simulink library "lib_HVESS"  (R2017a)
settings: Solver=VariableStepAuto  StartTime=0.0  StopTime=10.0  RelTol=1e-3
undefined symbols (not defined in the file): Atm_temp, bms_inletair_temp, bms_maxchargecurrent, bms_maxdischargecurrent, BMS_Notfallkuehlung, Cells, Chg, Em, ess, I_loss, mph2kph, R_0, R_1, SOC_bp, T_bp, tloop
libraries: fl_lib x13, simulink x9, nesl_utility x8, RollingAliveCounter x1
(part 1 of 2)
settings Model: Creator=Di Russo  LastModifiedBy=Vraj M

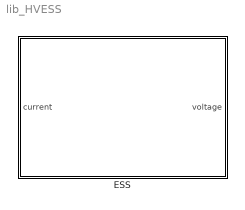
== system lib_HVESS ==
  ESS : Subsystem
      mask Display:
      | image('Images/ESS.jpg')
      | color('red');
      | port_label('Input',1,'Crr');
      | port_label('Output',1,'Volt');

== system lib_HVESS/ESS ==
  note: BMS_to_Actuators
  current : Inport
  ESS : Subsystem
      mask Display:
      | image('Images/ESS.jpg')
      | color('red');
      | port_label('Input',2,'Crr');
      | port_label('Output',2,'Volt');
  Inputs : Subsystem
  Outputs : Subsystem
  Soft BMS : Subsystem  RequirementInfo={} %GIDa_db9a4bec_736d_475e_b698_7a828f195e96
      mask Display: image('SoftECU.jpg')
  voltage : Outport
  wires:
  Inputs/1(Inputs) -> Soft BMS/1(Input1)
  Soft BMS/1(CAN) -> Outputs/1(Outputs)
  ESS/2(Voltage) -> voltage/1
  ESS/1(out) -> Soft BMS/2(Input2)  "Sensors_to_BMS"
  Soft BMS/2(Output2) -> ESS/1("In ")
  current/1 -> ESS/2("Crr ")

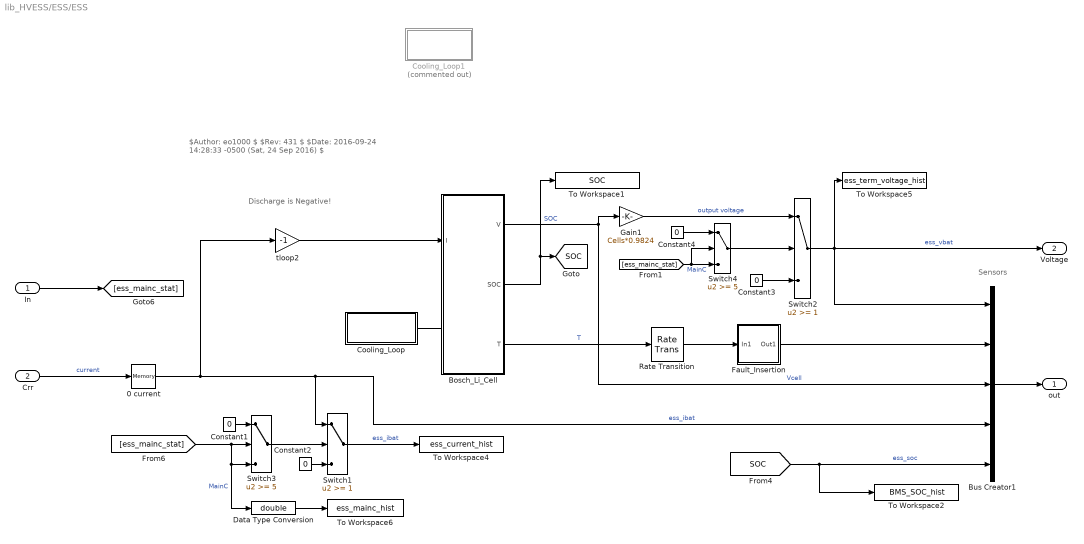
== system lib_HVESS/ESS/ESS ==
  note: $Author: eo1000 $
      | $Rev: 431 $
      | $Date: 2016-09-24 14:28:33 -0500 (Sat, 24 Sep 2016) $
  note: Discharge is Negative!
  note: Sensors
  "In " : Inport
  "Crr " : Inport  Port=2
  0 current : Memory  InheritSampleTime=on
  Bosch_Li_Cell : Subsystem
  Bus Creator1 : BusCreator  Inputs=5
  Constant{1..4} (4 alike) : Constant  Value=0
  Cooling_Loop : Subsystem
  Cooling_Loop1 : Subsystem  Commented=on
  Data Type Conversion : DataTypeConversion  OutDataTypeStr=double
  Fault_Insertion : Subsystem
  Gain1 : Gain  Gain=Cells*0.9824
  Rate Transition : RateTransition  X0=273.15+25
  Switch1 : Switch  Threshold=1
  Switch2 : Switch  Threshold=1
  Switch3 : Switch  Threshold=5
  Switch4 : Switch  Threshold=5
  To Workspace1 : ToWorkspace  VariableName=SOC  SampleTime=-1
      settings: Decimation=WORKSPACE_DECIMATION
  To Workspace2 : ToWorkspace  VariableName=BMS_SOC_hist  SampleTime=-1
      settings: Decimation=WORKSPACE_DECIMATION
  To Workspace4 : ToWorkspace  VariableName=ess_current_hist  SampleTime=-1
      settings: Decimation=WORKSPACE_DECIMATION
  To Workspace5 : ToWorkspace  VariableName=ess_term_voltage_hist  SampleTime=-1
      settings: Decimation=WORKSPACE_DECIMATION
  To Workspace6 : ToWorkspace  VariableName=ess_mainc_hist  SampleTime=-1
      settings: Decimation=WORKSPACE_DECIMATION
  tloop2 : Gain  Gain=-1
  out : Outport
  Voltage : Outport  Port=2
  tag scope: SOC=global
  wires:
  Rate Transition/1 -> Fault_Insertion/1(In1)
  Fault_Insertion/1(Out1) -> Bus Creator1/2
  tloop2/1 -> Bosch_Li_Cell/1(I)
  Bosch_Li_Cell/2(SOC) -> [SOC], To Workspace1/1  "SOC"
  Bosch_Li_Cell/3(T) -> Rate Transition/1  "T"
  "Crr "/1 -> 0 current/1  "current"
  0 current/1 -> Switch1/1, Bus Creator1/4, tloop2/1  "ess_ibat"
  Switch4/1 -> Switch2/2
  Constant4/1 -> Switch4/1
  [ess_mainc_stat] -> Switch4/2, Switch4/3  "MainC"
  Switch3/1 -> Switch1/2
  Constant1/1 -> Switch3/1
  Bosch_Li_Cell/1(V) -> Bus Creator1/3, Gain1/1  "Vcell"
  [SOC] -> Bus Creator1/5, To Workspace2/1  "ess_soc"
  Switch2/1 -> To Workspace5/1, Voltage/1, Bus Creator1/1  "ess_vbat"
  Constant3/1 -> Switch2/3
  [ess_mainc_stat] -> Switch3/2, Switch3/3, Data Type Conversion/1  "MainC"
  Gain1/1 -> Switch2/1  "output voltage"
  Switch1/1 -> To Workspace4/1  "ess_ibat"
  Constant2/1 -> Switch1/3
  Data Type Conversion/1 -> To Workspace6/1
  Bus Creator1/1 -> out/1
  "In "/1 -> [ess_mainc_stat]
  connections:
  Cooling_Loop/RConn1 -- Bosch_Li_Cell/LConn1

== system lib_HVESS/ESS/Inputs ==
  Bus Creator1 : BusCreator  Inputs=2
  CAN_fromHCU : Subsystem
  Digital_fromHCU : Subsystem
  Inputs : Outport
  wires:
  Bus Creator1/1 -> Inputs/1
  CAN_fromHCU/1(Outputs) -> Bus Creator1/1  "CAN"
  Digital_fromHCU/1(Outputs) -> Bus Creator1/2  "Digital"

== system lib_HVESS/ESS/Outputs ==
  Outputs : Inport
  tag scope: BMS_to_HCU=global
  wires:
  Outputs/1 -> [BMS_to_HCU]  "BMS_CAN"

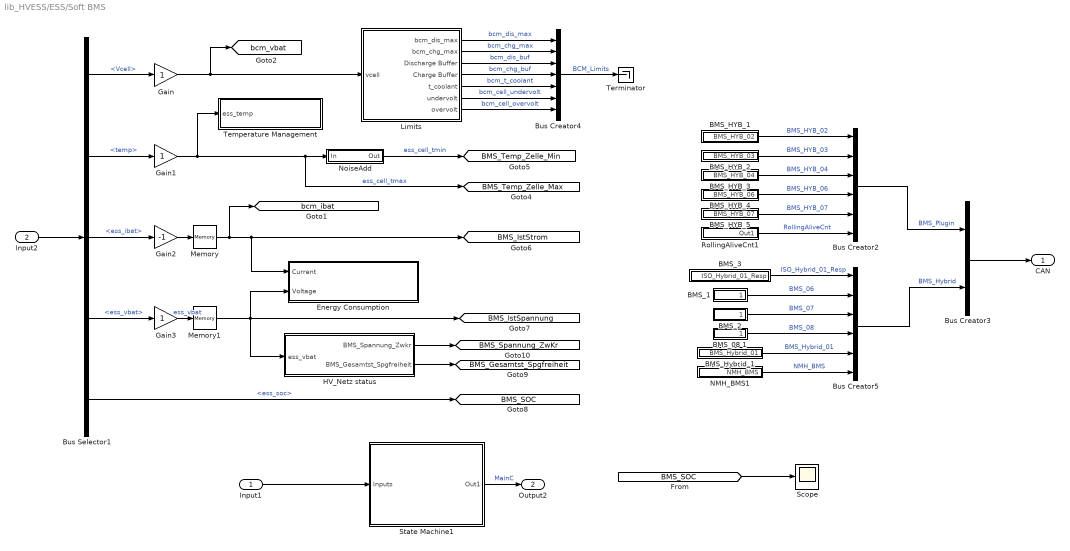
== system lib_HVESS/ESS/Soft BMS ==
  Input1 : Inport
  Input2 : Inport  Port=2
  BMS_08 1 : Subsystem
  BMS_1 : Subsystem
  BMS_2 : Subsystem
  BMS_3 : Subsystem
  BMS_HYB_1 : Subsystem
  BMS_HYB_2 : Subsystem
  BMS_HYB_3 : Subsystem
  BMS_HYB_4 : Subsystem
  BMS_HYB_5 : Subsystem
  BMS_Hybrid_1 : Subsystem
  Bus Creator2 : BusCreator  Inputs=6
  Bus Creator3 : BusCreator  Inputs=2
  Bus Creator4 : BusCreator  Inputs=7
  Bus Creator5 : BusCreator  Inputs=6
  Bus Selector1 : BusSelector  OutputSignals=Vcell,temp,ess_ibat,ess_vbat,ess_soc
  Energy Consumption : Subsystem
  Gain : Gain
  Gain1 : Gain
  Gain2 : Gain  Gain=-1
  Gain3 : Gain
  HV_Netz status : Subsystem
  Limits : Subsystem
  Memory : Memory
  Memory1 : Memory
  NMH_BMS1 : Subsystem
  NoiseAdd : Subsystem
  RollingAliveCnt1 : Subsystem
  Scope : Scope
  State Machine1 : Subsystem
  Temperature Management : Subsystem
  Terminator : Terminator
  CAN : Outport
  Output2 : Outport  Port=2
  tag scope: BMS_Gesamtst_Spgfreiheit=global, BMS_IstSpannung=global, BMS_IstStrom=global, BMS_SOC=global, BMS_Spannung_ZwKr=global, BMS_Temp_Zelle_Max=global, BMS_Temp_Zelle_Min=global, bcm_ibat=global, bcm_vbat=global
  wires:
  [BMS_SOC] -> Scope/1
  RollingAliveCnt1/1(Out1) -> Bus Creator2/6  "RollingAliveCnt"
  BMS_3/1(ISO_Hybrid_01_Resp) -> Bus Creator5/1  "ISO_Hybrid_01_Resp"
  Bus Creator2/1 -> Bus Creator3/1  "BMS_Plugin"
  Bus Creator5/1 -> Bus Creator3/2  "BMS_Hybrid"
  BMS_08 1/1(BMS_08) -> Bus Creator5/4  "BMS_08"
  BMS_1/1(BMS_06) -> Bus Creator5/2  "BMS_06"
  BMS_HYB_4/1(BMS_HYB_06) -> Bus Creator2/4  "BMS_HYB_06"
  BMS_HYB_1/1(BMS_HYB_02) -> Bus Creator2/1  "BMS_HYB_02"
  BMS_HYB_3/1(BMS_HYB_04) -> Bus Creator2/3  "BMS_HYB_04"
  BMS_2/1(BMS_07) -> Bus Creator5/3  "BMS_07"
  BMS_Hybrid_1/1(BMS_Hybrid_01) -> Bus Creator5/5  "BMS_Hybrid_01"
  BMS_HYB_5/1(BMS_HYB_07) -> Bus Creator2/5  "BMS_HYB_07"
  BMS_HYB_2/1(BMS_HYB_03) -> Bus Creator2/2  "BMS_HYB_03"
  NMH_BMS1/1(NMH_BMS) -> Bus Creator5/6  "NMH_BMS"
  Memory1/1 -> Energy Consumption/2(Voltage), HV_Netz status/1(ess_vbat), [BMS_IstSpannung]
  Memory/1 -> [BMS_IstStrom], Energy Consumption/1(Current), [bcm_ibat]
  HV_Netz status/2(BMS_Gesamtst_Spgfreiheit) -> [BMS_Gesamtst_Spgfreiheit]
  HV_Netz status/1(BMS_Spannung_Zwkr) -> [BMS_Spannung_ZwKr]
  Bus Creator3/1 -> CAN/1
  Limits/7(overvolt) -> Bus Creator4/7  "bcm_cell_overvolt"
  Limits/6(undervolt) -> Bus Creator4/6  "bcm_cell_undervolt"
  Bus Selector1/4 -> Gain3/1  "<ess_vbat>"
  Bus Selector1/5 -> [BMS_SOC]  "<ess_soc>"
  Bus Creator4/1 -> Terminator/1  "BCM_Limits"
  Limits/2(bcm_chg_max) -> Bus Creator4/2  "bcm_chg_max"
  Limits/5(t_coolant) -> Bus Creator4/5  "bcm_t_coolant"
  Limits/4(Charge Buffer) -> Bus Creator4/4  "bcm_chg_buf"
  Limits/3(Discharge Buffer) -> Bus Creator4/3  "bcm_dis_buf"
  Limits/1(bcm_dis_max) -> Bus Creator4/1  "bcm_dis_max"
  Gain1/1 -> [BMS_Temp_Zelle_Max], NoiseAdd/1(In), Temperature Management/1(ess_temp)  "ess_cell_tmax"
  Bus Selector1/2 -> Gain1/1  "<temp>"
  Bus Selector1/1 -> Gain/1  "<Vcell>"
  NoiseAdd/1(Out) -> [BMS_Temp_Zelle_Min]  "ess_cell_tmin"
  Bus Selector1/3 -> Gain2/1  "<ess_ibat>"
  Input2/1 -> Bus Selector1/1
  Input1/1 -> State Machine1/1(Inputs)
  Gain/1 -> Limits/1(vcell), [bcm_vbat]
  Gain2/1 -> Memory/1
  Gain3/1 -> Memory1/1  "ess_vbat"
  State Machine1/1(Out1) -> Output2/1  "MainC"

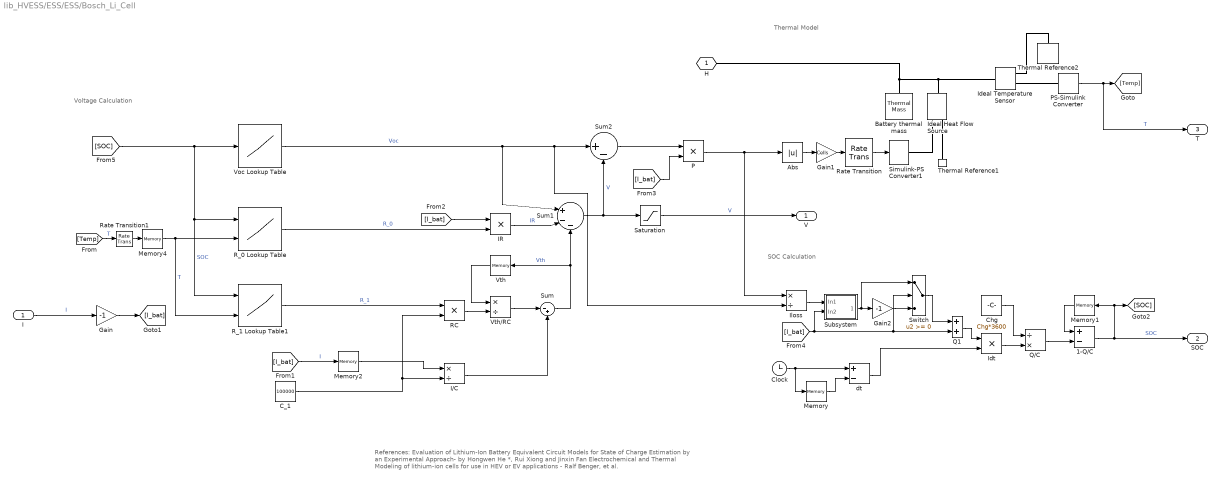
== system lib_HVESS/ESS/ESS/Bosch_Li_Cell ==
  note: SOC Calculation
  note: Thermal Model
  note: Voltage Calculation
  note: References:
      | Evaluation of Lithium-Ion Battery Equivalent Circuit Models for State of Charge Estimation by an Experimental Approach- by Hongwen He *, Rui Xiong and Jinxin Fan
      | Electrochemical and Thermal Modeling of lithium-ion cells for use in HEV or EV applications - Ralf Benger, et al.
  I : Inport
  1-Q/C : Sum  Inputs=+-
  Abs : Abs
  Battery thermal mass : fl_lib/Thermal/Thermal Elements/Thermal Mass  mass=155 kg  sp_heat=800 J/kg/K  T_specify=off  T_priority=High  T=Atm_temp degC  T_nominal_specify=off  T_nominal_unit=K  T_nominal_value=1  Q_specify=off  Q_priority=High  Q=0 J/s  Q_nominal_specify=off  Q_nominal_unit=J/s  Q_nominal_value=1
  C_1 : Constant  Value=100000
  Chg : Constant  Value=Chg*3600
  Clock : Clock
  Gain : Gain  Gain=-1
  Gain1 : Gain  Gain=Cells
  Gain2 : Gain  Gain=-1
  I/C : Product  Inputs=*/
  IR : Product  Inputs=**
  Ideal Heat Flow Source : fl_lib/Thermal/Thermal Sources/Ideal Heat Flow Source
      settings: SourceProductName=Simscape  SourceProductBaseCode=SS
  Ideal Temperature Sensor : fl_lib/Thermal/Thermal Sensors/Ideal Temperature Sensor
      settings: SourceProductName=Simscape  SourceProductBaseCode=SS
  Idt : Product  Inputs=**
  Iloss : Product  Inputs=*/
  Memory : Memory  InheritSampleTime=on
  Memory1 : Memory  X0=ess.plant.initial_soc/100  InheritSampleTime=on
  Memory2 : Memory  InheritSampleTime=on
  Memory4 : Memory  X0=298
  P : Product  Inputs=**
  PS-Simulink Converter : nesl_utility/PS-Simulink Converter  PhysicalDomain=network_engine_domain  SubClassName=ps_output  LeftPortType=input  RightPortType=output  PseudoPeriodic=off  Frequencies=[]  Unit=1  AffineConversion=off
  Q/C : Product  Inputs=/*
  Q1 : Sum
  RC : Product  Inputs=**
  R_0 Lookup Table : Lookup_n-D  BreakpointsForDimension1=SOC_bp  BreakpointsForDimension2=T_bp  Table=R_0  UseLastTableValue=on  InternalRulePriority=Speed  RndMeth=Simplest  InputSameDT=on
  R_1 Lookup Table1 : Lookup_n-D  BreakpointsForDimension1=SOC_bp  BreakpointsForDimension2=T_bp  Table=R_1  UseLastTableValue=on  InternalRulePriority=Speed  RndMeth=Simplest  InputSameDT=on
  Rate Transition : RateTransition
  Rate Transition1 : RateTransition
  Saturation : Saturate  UpperLimit=4.2  LowerLimit=2.8
  Simulink-PS Converter1 : nesl_utility/Simulink-PS Converter  PhysicalDomain=network_engine_domain  SubClassName=ps_input  LeftPortType=input  RightPortType=output  PseudoPeriodic=off  Frequencies=[]  NoiseDistribution=none  NoiseParameters=[]  Unit=1  AffineConversion=off  FilteringAndDerivatives=zero  SimscapeFilterOrder=1  InputFilterTimeConstant=0.001  UdotUserProvided=1
  Subsystem : Subsystem
  Sum : Sum  Inputs=|-+
  Sum1 : Sum  Inputs=|+--
  Sum2 : Sum  Inputs=|+-
  Switch : Switch
  Thermal Reference1 : fl_lib/Thermal/Thermal Elements/Thermal Reference
  Thermal Reference2 : fl_lib/Thermal/Thermal Elements/Thermal Reference
  Voc Lookup Table : Lookup_n-D  NumberOfTableDimensions=1  BreakpointsForDimension1=SOC_bp  Table=Em  InternalRulePriority=Speed  RndMeth=Simplest  InputSameDT=on
  Vth : Memory  InheritSampleTime=on  LinearizeAsDelay=on
  Vth/RC : Product  Inputs=*/
  dt : Sum  Inputs=+-
  H : PMIOPort  Tag=PMCPort  Port=1  Side=Left
  V : Outport
  SOC : Outport  Port=2
  T : Outport  Port=3
  wires:
  Rate Transition1/1 -> Memory4/1
  Subsystem/1(Out1) -> Gain2/1, Switch/1
  Iloss/1 -> Subsystem/1(In1)
  Switch/1 -> Q1/1
  Q1/1 -> Idt/1
  Gain2/1 -> Switch/3
  Gain1/1 -> Rate Transition/1
  P/1 -> Abs/1, Iloss/1
  Memory2/1 -> I/C/1
  Idt/1 -> Q/C/2
  dt/1 -> Idt/2
  Memory/1 -> dt/2
  Clock/1 -> dt/1, Memory/1
  Gain/1 -> [I_bat]
  Memory1/1 -> 1-Q/C/1
  Q/C/1 -> 1-Q/C/2
  Chg/1 -> Q/C/1
  1-Q/C/1 -> [SOC], Memory1/1, SOC/1  "SOC"
  Memory4/1 -> R_0 Lookup Table/2, R_1 Lookup Table1/2  "T"
  Saturation/1 -> V/1  "V"
  I/1 -> Gain/1  "I"
  Voc Lookup Table/1 -> Sum1/1, Sum2/1, Iloss/2  "Voc"
  R_1 Lookup Table1/1 -> RC/1  "R_1"
  PS-Simulink Converter/1 -> [Temp], T/1  "T"
  [I_bat] -> P/2
  [I_bat] -> IR/1
  Sum1/1 -> Sum2/2, Saturation/1  "V"
  Vth/1 -> Vth/RC/1
  I/C/1 -> Sum/2
  [I_bat] -> Memory2/1  "I"
  RC/1 -> Vth/RC/2
  C_1/1 -> I/C/2, RC/2
  Sum2/1 -> P/1
  Sum/1 -> Vth/1, Sum1/3  "Vth"
  IR/1 -> Sum1/2  "IR"
  [SOC] -> Voc Lookup Table/1, R_1 Lookup Table1/1, R_0 Lookup Table/1  "SOC"
  [Temp] -> Rate Transition1/1  "T"
  Rate Transition/1 -> Simulink-PS Converter1/1
  Abs/1 -> Gain1/1
  [I_bat] -> Switch/2, Q1/2, Subsystem/2(In2)
  R_0 Lookup Table/1 -> IR/2  "R_0"
  Vth/RC/1 -> Sum/1
  connections:
  Ideal Heat Flow Source/RConn1 -- Simulink-PS Converter1/RConn1
  Ideal Temperature Sensor/RConn2 -- PS-Simulink Converter/LConn1
  Ideal Temperature Sensor/RConn1 -- Thermal Reference2/LConn1
  Ideal Heat Flow Source/RConn2 -- Thermal Reference1/LConn1
  Ideal Heat Flow Source/LConn1 -- Battery thermal mass/LConn1 -- H/RConn1 -- Ideal Temperature Sensor/LConn1

== system lib_HVESS/ESS/ESS/Cooling_Loop ==
  Constant : Constant  Value=Atm_temp+273+0.5
  Convective Heat Transfer : fl_lib/Thermal/Thermal Elements/Convective Heat Transfer  area=1e-4*Cells*0.25 m^2  heat_tr_coeff=H_coef W/(m^2 * K)  Q_specify=off  Q_priority=High  Q=0 J/s  Q_nominal_specify=off  Q_nominal_unit=J/s  Q_nominal_value=1  T_specify=off  T_priority=High  T=0 K  T_nominal_specify=off  T_nominal_unit=K  T_nominal_value=1
  Ideal Temperature Source : fl_lib/Thermal/Thermal Sources/Ideal Temperature Source
      settings: SourceProductName=Simscape  SourceProductBaseCode=SS
  Simulink-PS Converter : nesl_utility/Simulink-PS Converter  PhysicalDomain=network_engine_domain  SubClassName=ps_input  LeftPortType=input  RightPortType=output  PseudoPeriodic=off  Frequencies=[]  NoiseDistribution=none  NoiseParameters=[]  Unit=1  AffineConversion=off  FilteringAndDerivatives=zero  SimscapeFilterOrder=1  InputFilterTimeConstant=0.001  UdotUserProvided=1
  Solver Configuration : nesl_utility/Solver Configuration  PhysicalDomain=network_engine_domain  SubClassName=solver  LeftPortType=input  RightPortType=generic  Accelerate=off  Tones=[]  Harmonics=[]  SimulateNoise=off  Profile=off  UseLocalSampling=off  EnableSwitchedLinearOptims=on  FrequencyDomain=off  UseCCode=off  RelTol=0.001  AbsTol=1e-06  MinStep=1e-09  ToWorkspace=off  RevertToSquareIcSolve=off  NumHomotopyIterations=100  PhasorMode=off  PhasorModeNumHarmonics=1  OverrideAbsTol=off  DoDC=off  ResidualTolerance=1e-09  UseLocalSolver=on  LocalSolverChoice=NE_TRAPEZOIDAL_ADVANCER  LocalSolverSampleTime=1  DoFixedCost=on  MaxNonlinIter=3  MaxModeIter=2  LinearAlgebra=Sparse  DelaysMemoryBudget=1024  AutomaticFiltering=on  FilteringTimeConstant=0.001
  Thermal Reference : fl_lib/Thermal/Thermal Elements/Thermal Reference
  Conn1 : PMIOPort  Port=1  Side=Right
  wires:
  Constant/1 -> Simulink-PS Converter/1
  connections:
  Conn1/RConn1 -- Solver Configuration/RConn1 -- Convective Heat Transfer/LConn1
  Ideal Temperature Source/RConn1 -- Simulink-PS Converter/RConn1
  Ideal Temperature Source/LConn1 -- Convective Heat Transfer/RConn1
  Ideal Temperature Source/RConn2 -- Thermal Reference/LConn1

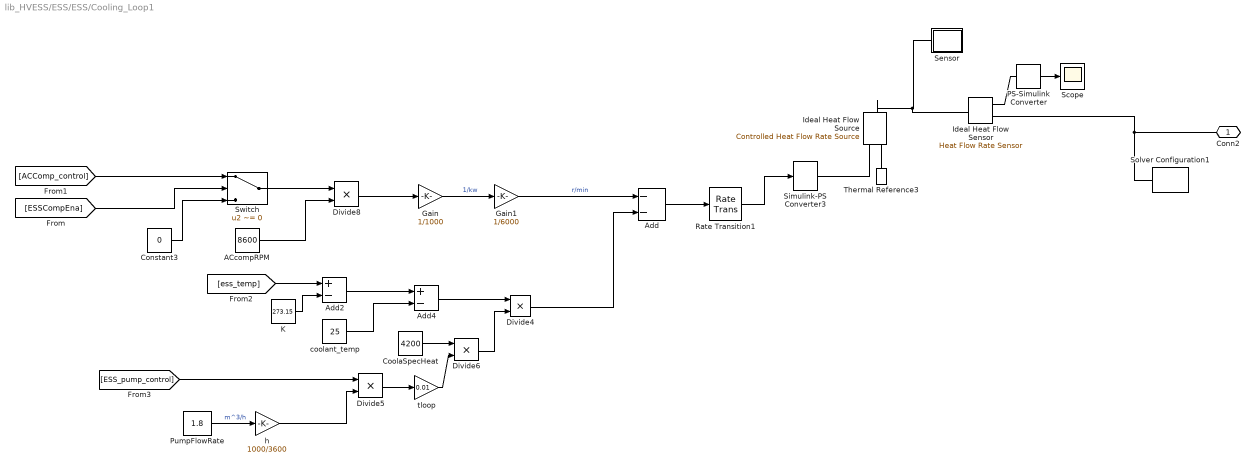
== system lib_HVESS/ESS/ESS/Cooling_Loop1 ==
  ACcompRPM : Constant  Value=8600
  Add : Sum  Inputs=--
  Add2 : Sum  Inputs=+-
  Add4 : Sum  Inputs=+-
  Constant3 : Constant  Value=0
  CoolaSpecHeat : Constant  Value=4200
  Divide{4..6,8} (4 alike) : Product  Inputs=**
  Gain : Gain  Gain=1/1000
  Gain1 : Gain  Gain=1/6000
  Ideal Heat Flow Sensor : fl_lib/Thermal/Thermal Sensors/Heat Flow Rate Sensor
      settings: SourceProductName=Simscape  SourceProductBaseCode=SS
  Ideal Heat Flow Source : fl_lib/Thermal/Thermal Sources/Controlled Heat Flow Rate Source
      settings: SourceProductName=Simscape
  K : Constant  Value=273.15
  PS-Simulink Converter : nesl_utility/PS-Simulink Converter  PhysicalDomain=network_engine_domain  SubClassName=ps_output  LeftPortType=input  RightPortType=output  PseudoPeriodic=off  Frequencies=[]  Unit=1  AffineConversion=off
  PumpFlowRate : Constant  Value=1.8
  Rate Transition1 : RateTransition
  Scope : Scope
  Sensor : Subsystem
  Simulink-PS Converter3 : nesl_utility/Simulink-PS Converter  PhysicalDomain=network_engine_domain  SubClassName=ps_input  LeftPortType=input  RightPortType=output  PseudoPeriodic=off  Frequencies=[]  NoiseDistribution=none  NoiseParameters=[]  Unit=J/s  AffineConversion=off  FilteringAndDerivatives=zero  SimscapeFilterOrder=1  InputFilterTimeConstant=0.001  UdotUserProvided=1
  Solver Configuration1 : nesl_utility/Solver Configuration  PhysicalDomain=network_engine_domain  SubClassName=solver  LeftPortType=input  RightPortType=generic  Accelerate=off  Tones=[]  Harmonics=[]  SimulateNoise=off  Profile=off  UseLocalSampling=off  EnableSwitchedLinearOptims=on  FrequencyDomain=off  UseCCode=off  RelTol=0.001  AbsTol=1e-06  MinStep=1e-09  ToWorkspace=off  RevertToSquareIcSolve=off  NumHomotopyIterations=100  PhasorMode=off  PhasorModeNumHarmonics=1  OverrideAbsTol=off  DoDC=off  ResidualTolerance=1e-09  UseLocalSolver=on  LocalSolverChoice=NE_BACKWARD_EULER_ADVANCER  LocalSolverSampleTime=1  DoFixedCost=on  MaxNonlinIter=3  MaxModeIter=2  LinearAlgebra=Sparse  DelaysMemoryBudget=1024  AutomaticFiltering=on  FilteringTimeConstant=0.001
  Switch : Switch  Criteria=u2 ~= 0
  Thermal Reference3 : fl_lib/Thermal/Thermal Elements/Thermal Reference
  coolant_temp : Constant  Value=25
  h : Gain  Gain=1000/3600
  tloop : Gain  Gain=0.01
  Conn2 : PMIOPort  Port=1  Side=Left
  wires:
  PS-Simulink Converter/1 -> Scope/1
  [ESS_pump_control] -> Divide5/1
  Switch/1 -> Divide8/1
  Add/1 -> Rate Transition1/1
  Rate Transition1/1 -> Simulink-PS Converter3/1
  K/1 -> Add2/2
  [ess_temp] -> Add2/1
  Add2/1 -> Add4/1
  Constant3/1 -> Switch/3
  Divide4/1 -> Add/2
  PumpFlowRate/1 -> h/1  "m^3/h"
  Divide5/1 -> tloop/1
  ACcompRPM/1 -> Divide8/2
  Gain1/1 -> Add/1  "r/min"
  [ACComp_control] -> Switch/1
  Gain/1 -> Gain1/1  "1/kw"
  h/1 -> Divide5/2
  coolant_temp/1 -> Add4/2
  CoolaSpecHeat/1 -> Divide6/1
  Add4/1 -> Divide4/1
  Divide8/1 -> Gain/1
  tloop/1 -> Divide6/2
  Divide6/1 -> Divide4/2
  [ESSCompEna] -> Switch/2
  connections:
  Ideal Heat Flow Sensor/RConn1 -- PS-Simulink Converter/LConn1
  Conn2/RConn1 -- Ideal Heat Flow Sensor/RConn2 -- Solver Configuration1/RConn1
  Thermal Reference3/LConn1 -- Ideal Heat Flow Source/RConn2
  Simulink-PS Converter3/RConn1 -- Ideal Heat Flow Source/RConn1
  Sensor/LConn1 -- Ideal Heat Flow Sensor/LConn1 -- Ideal Heat Flow Source/LConn1

== system lib_HVESS/ESS/ESS/Fault_Insertion ==
  In1 : Inport
  Gain : Gain  Gain=3
  Switch : Switch  Threshold=1
  Out1 : Outport
  wires:
  Gain/1 -> Switch/1
  Switch/1 -> Out1/1  "temp"
  In1/1 -> Switch/3, Gain/1
  [ESSOverTemp] -> Switch/2

== system lib_HVESS/ESS/Inputs/CAN_fromHCU ==
  Bus Creator : BusCreator  Inputs=2
  Outputs : Outport
  wires:
  Bus Creator/1 -> Outputs/1
  [HCU_to_EBCAN] -> Bus Creator/2
  [HCU_to_HV_CAN] -> Bus Creator/1

== system lib_HVESS/ESS/Inputs/Digital_fromHCU ==
  Outputs : Outport
  wires:
  [Digital] -> Outputs/1

== system lib_HVESS/ESS/Soft BMS/BMS_08 1 ==
  Bus Creator8 : BusCreator  Inputs=2
  BMS_08 : Outport
  wires:
  [BMS_Temp_Zelle_Max] -> Bus Creator8/1  "BMS_Temp_Zelle_Max"
  Bus Creator8/1 -> BMS_08/1  "BMS_08"
  [BMS_Temp_Zelle_Min] -> Bus Creator8/2  "BMS_Temp_Zelle_Min"

== system lib_HVESS/ESS/Soft BMS/BMS_1 ==
  Bus Creator8 : BusCreator  Inputs=1
  Constant2 : Constant  Value=0
  BMS_06 : Outport
  wires:
  Constant2/1 -> Bus Creator8/1  "BMS_SollVolumenStrom"
  Bus Creator8/1 -> BMS_06/1  "BMS_06"

== system lib_HVESS/ESS/Soft BMS/BMS_2 ==
  Bus Creator8 : BusCreator  Inputs=1
  BMS_07 : Outport
  wires:
  [BMS_Gesamtst_Spgfreiheit] -> Bus Creator8/1  "BMS_Gesamtst_Spgfreiheit"
  Bus Creator8/1 -> BMS_07/1  "BMS_07"

== system lib_HVESS/ESS/Soft BMS/BMS_3 ==
  Bus Creator8 : BusCreator  Inputs=3
  Constant : Constant  Value=255
  Constant1 : Constant  Value=254
  Data Type Conversion : DataTypeConversion
  ISO_Hybrid_01_Resp : Outport
  wires:
  [ISO_Hybrid_01_Req_Data_4] -> Data Type Conversion/1  "ISO_Hybrid_01_Resp_Data_4"
  Constant1/1 -> Bus Creator8/3  "ISO_Hybrid_01_Resp_Data_6"
  Constant/1 -> Bus Creator8/2  "ISO_Hybrid_01_Resp_Data_5"
  Data Type Conversion/1 -> Bus Creator8/1  "ISO_Hybrid_01_Resp_Data_4"
  Bus Creator8/1 -> ISO_Hybrid_01_Resp/1  "ISO_Hybrid_01_Resp"

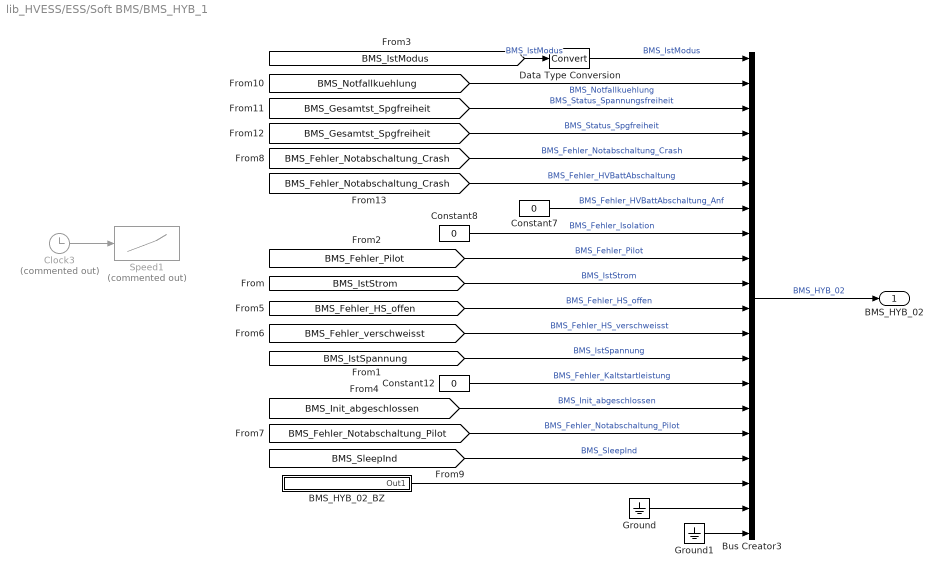
== system lib_HVESS/ESS/Soft BMS/BMS_HYB_1 ==
  BMS_HYB_02_BZ : Subsystem
  Bus Creator3 : BusCreator  Inputs=20
  Clock3 : Clock  Commented=on
  Constant12 : Constant  Value=0
  Constant7 : Constant  Value=0
  Constant8 : Constant  Value=0
  Data Type Conversion : DataTypeConversion
  Ground : Ground
  Ground1 : Ground
  Speed1 : Lookup  Commented=on  InputValues=[0 75 75 100 100 120]  Table=[0 0 1 1 0 0]
  BMS_HYB_02 : Outport
  wires:
  Ground1/1 -> Bus Creator3/20
  Ground/1 -> Bus Creator3/19
  BMS_HYB_02_BZ/1(Out1) -> Bus Creator3/18
  [BMS_IstModus] -> Data Type Conversion/1  "BMS_IstModus"
  Clock3/1 -> Speed1/1
  Bus Creator3/1 -> BMS_HYB_02/1  "BMS_HYB_02"
  Data Type Conversion/1 -> Bus Creator3/1  "BMS_IstModus"
  [BMS_Gesamtst_Spgfreiheit] -> Bus Creator3/3  "BMS_Status_Spannungsfreiheit"
  [BMS_Fehler_Notabschaltung_Crash] -> Bus Creator3/6  "BMS_Fehler_HVBattAbschaltung"
  Constant7/1 -> Bus Creator3/7  "BMS_Fehler_HVBattAbschaltung_Anf"
  [BMS_Notfallkuehlung] -> Bus Creator3/2  "BMS_Notfallkuehlung"
  Constant8/1 -> Bus Creator3/8  "BMS_Fehler_Isolation"
  [BMS_Fehler_Notabschaltung_Crash] -> Bus Creator3/5  "BMS_Fehler_Notabschaltung_Crash"
  [BMS_Gesamtst_Spgfreiheit] -> Bus Creator3/4  "BMS_Status_Spgfreiheit"
  [BMS_Fehler_Pilot] -> Bus Creator3/9  "BMS_Fehler_Pilot"
  [BMS_IstStrom] -> Bus Creator3/10  "BMS_IstStrom"
  [BMS_Fehler_HS_offen] -> Bus Creator3/11  "BMS_Fehler_HS_offen"
  [BMS_Fehler_verschweisst] -> Bus Creator3/12  "BMS_Fehler_HS_verschweisst"
  [BMS_IstSpannung] -> Bus Creator3/13  "BMS_IstSpannung"
  Constant12/1 -> Bus Creator3/14  "BMS_Fehler_Kaltstartleistung"
  [BMS_Init_abgeschlossen] -> Bus Creator3/15  "BMS_Init_abgeschlossen"
  [BMS_Fehler_Notabschaltung_Pilot] -> Bus Creator3/16  "BMS_Fehler_Notabschaltung_Pilot"
  [BMS_SleepInd] -> Bus Creator3/17  "BMS_SleepInd"

== system lib_HVESS/ESS/Soft BMS/BMS_HYB_2 ==
  Bus Creator3 : BusCreator  Inputs=1
  Data Type Conversion : DataTypeConversion
  Gain : Gain  Gain=100
  BMS_HYB_03 : Outport
  wires:
  Gain/1 -> Data Type Conversion/1
  [BMS_SOC] -> Gain/1  "BMS_SOC"
  Data Type Conversion/1 -> Bus Creator3/1  "BMS_SOC"
  Bus Creator3/1 -> BMS_HYB_03/1  "BMS_HYB_03"

== system lib_HVESS/ESS/Soft BMS/BMS_HYB_3 ==
  Bus Creator6 : BusCreator  Inputs=3
  Constant : Constant
  Constant1 : Constant  Commented=on  Value=bms_maxdischargecurrent
  Constant2 : Constant
  Constant3 : Constant  Commented=on  Value=bms_maxchargecurrent
  BMS_HYB_04 : Outport
  wires:
  Constant/1 -> Bus Creator6/1  "BMS_MaxDyn_LadeStrom"
  Bus Creator6/1 -> BMS_HYB_04/1  "BMS_HYB_04"
  [BMS_Spannung_ZwKr] -> Bus Creator6/3  "BMS_Spannung_ZwKr"
  Constant2/1 -> Bus Creator6/2

== system lib_HVESS/ESS/Soft BMS/BMS_HYB_4 ==
  Bus Creator6 : BusCreator  Inputs=5
  Constant1 : Constant  Value=430
  Constant2 : Constant  Value=291
  Constant3 : Constant  Value=0
  Constant4 : Constant  Commented=on  Value=bms_inletair_temp
  Constant5 : Constant  Value=20
  BMS_HYB_06 : Outport
  wires:
  Constant1/1 -> Bus Creator6/2  "BMS_Max_LadeSpannung"
  Constant2/1 -> Bus Creator6/3  "BMS_Min_EntladeSpannung"
  Bus Creator6/1 -> BMS_HYB_06/1  "BMS_HYB_06"
  Constant3/1 -> Bus Creator6/1  "BMS_Balancing_Anf"
  [BMS_Temperatur] -> Bus Creator6/4  "BMS_Temperatur"
  Constant5/1 -> Bus Creator6/5  "BMS_Temperatur_Ansaugluft"

== system lib_HVESS/ESS/Soft BMS/BMS_HYB_5 ==
  Bus Creator6 : BusCreator  Inputs=1
  BMS_HYB_07 : Outport
  wires:
  [BMS_Temperierung_Anf] -> Bus Creator6/1  "BMS_Temperierung_Anf"
  Bus Creator6/1 -> BMS_HYB_07/1  "BMS_HYB_07"

== system lib_HVESS/ESS/Soft BMS/BMS_Hybrid_1 ==
  Bus Creator8 : BusCreator  Inputs=1
  BMS_Hybrid_01 : Outport
  wires:
  Bus Creator8/1 -> BMS_Hybrid_01/1  "BMS_Hybrid_01"
  [BMS_HYB_Kuehlung_Anf] -> Bus Creator8/1  "BMS_HYB_Kuehlung_Anf"

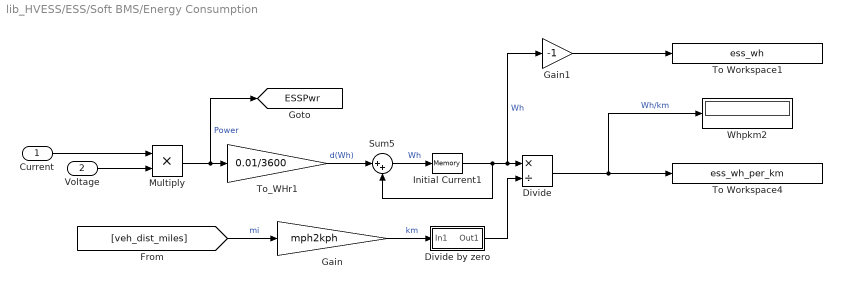
== system lib_HVESS/ESS/Soft BMS/Energy Consumption ==
  Current : Inport
  Voltage : Inport  Port=2
  Divide : Product  Inputs=*/
  Divide by zero : Subsystem
  Gain : Gain  Gain=mph2kph
  Gain1 : Gain  Gain=-1
  Initial Current1 : Memory  InheritSampleTime=on
  Multiply : Product  Inputs=**
  Sum5 : Sum  Inputs=|++  SaturateOnIntegerOverflow=on  InputSameDT=on  OutDataTypeStr=Inherit: Same as first input
  To Workspace1 : ToWorkspace  VariableName=ess_wh  SampleTime=-1
      settings: Decimation=WORKSPACE_DECIMATION
  To Workspace4 : ToWorkspace  VariableName=ess_wh_per_km  SampleTime=-1
      settings: Decimation=WORKSPACE_DECIMATION
  To_WHr1 : Gain  Gain=0.01/3600  SaturateOnIntegerOverflow=on  OutDataTypeStr=Inherit: Same as input  ParamDataTypeStr=Inherit: Same as input
  Whpkm2 : Display
  tag scope: ESSPwr=global
  wires:
  Gain1/1 -> To Workspace1/1
  Divide by zero/1(Out1) -> Divide/2
  Gain/1 -> Divide by zero/1(In1)  "km"
  Divide/1 -> To Workspace4/1, Whpkm2/1  "Wh/km"
  [veh_dist_miles] -> Gain/1  "mi"
  Initial Current1/1 -> Divide/1, Gain1/1, Sum5/2  "Wh"
  Sum5/1 -> Initial Current1/1  "Wh"
  To_WHr1/1 -> Sum5/1  "d(Wh)"
  Multiply/1 -> To_WHr1/1, [ESSPwr]  "Power"
  Voltage/1 -> Multiply/2
  Current/1 -> Multiply/1

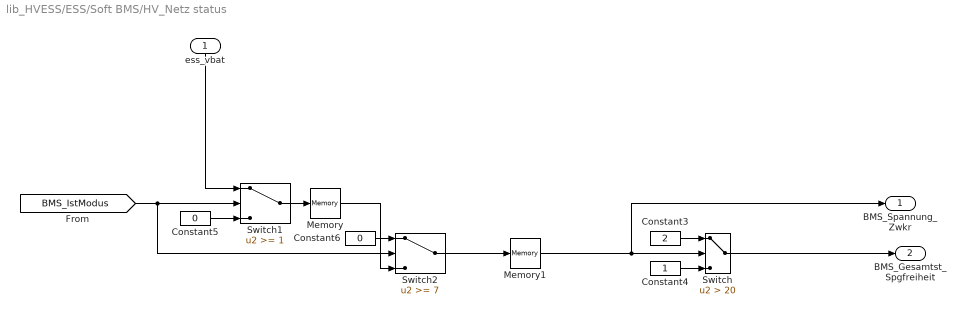
== system lib_HVESS/ESS/Soft BMS/HV_Netz status ==
  ess_vbat : Inport
  Constant3 : Constant  Value=2
  Constant4 : Constant
  Constant5 : Constant  Value=0
  Constant6 : Constant  Value=0
  Memory : Memory
  Memory1 : Memory
  Switch : Switch  Criteria=u2 > Threshold  Threshold=20
  Switch1 : Switch  Threshold=1
  Switch2 : Switch  Threshold=7
  BMS_Spannung_Zwkr : Outport
  BMS_Gesamtst_Spgfreiheit : Outport  Port=2
  wires:
  Memory1/1 -> Switch/2, BMS_Spannung_Zwkr/1
  Memory/1 -> Switch2/3
  ess_vbat/1 -> Switch1/1
  Constant3/1 -> Switch/1
  Switch/1 -> BMS_Gesamtst_Spgfreiheit/1
  Constant4/1 -> Switch/3
  Switch2/1 -> Memory1/1
  Constant6/1 -> Switch2/1
  Switch1/1 -> Memory/1
  [BMS_IstModus] -> Switch2/2, Switch1/2
  Constant5/1 -> Switch1/3

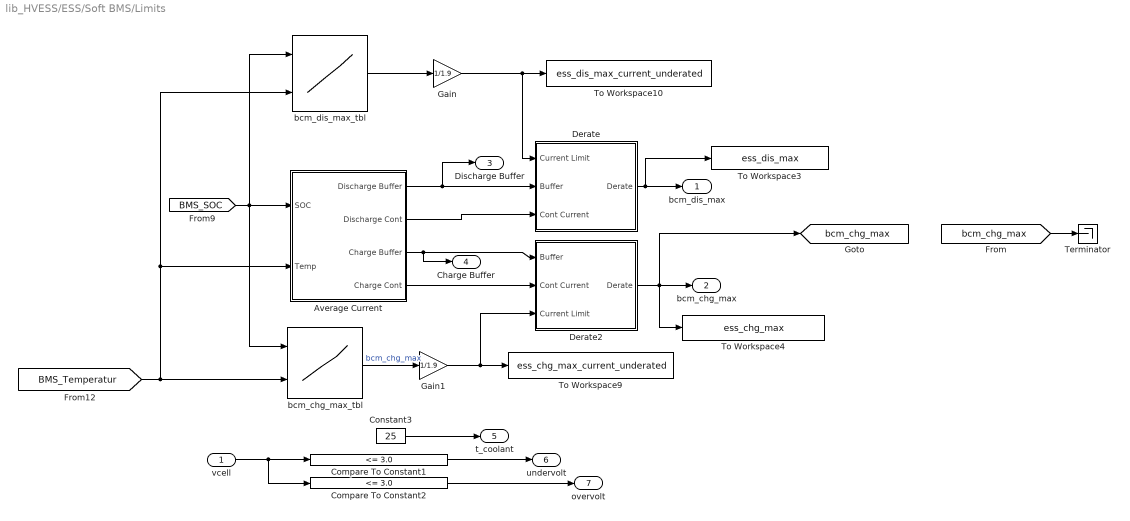
== system lib_HVESS/ESS/Soft BMS/Limits ==
  vcell : Inport
  Average Current : Subsystem
  Compare To Constant1 : simulink/Logic and Bit Operations/Compare To Constant  relop=<=  const=3.0  OutDataTypeStr=boolean
  Compare To Constant2 : simulink/Logic and Bit Operations/Compare To Constant  relop=<=  const=3.0  OutDataTypeStr=boolean
  Constant3 : Constant  Value=25
  Derate : Subsystem
  Derate2 : Subsystem
  Gain : Gain  Gain=1/1.9
  Gain1 : Gain  Gain=1/1.9
  Terminator : Terminator
  To Workspace10 : ToWorkspace  VariableName=ess_dis_max_current_underated  SampleTime=-1
      settings: Decimation=WORKSPACE_DECIMATION
  To Workspace3 : ToWorkspace  VariableName=ess_dis_max  SampleTime=-1
      settings: Decimation=WORKSPACE_DECIMATION
  To Workspace4 : ToWorkspace  VariableName=ess_chg_max  SampleTime=-1
      settings: Decimation=WORKSPACE_DECIMATION
  To Workspace9 : ToWorkspace  VariableName=ess_chg_max_current_underated  SampleTime=-1
      settings: Decimation=WORKSPACE_DECIMATION
  bcm_chg_max_tbl : Lookup2D  RowIndex=ess.plant.init.limit.idx1_soc  ColumnIndex=ess.plant.init.limit.idx2_temp  Table=ess.plant.init.max_charge_limit
  bcm_dis_max_tbl : Lookup2D  RowIndex=ess.plant.init.limit.idx1_soc  ColumnIndex=ess.plant.init.limit.idx2_temp  Table=ess.plant.init.max_discharge_limit
  bcm_dis_max : Outport
  bcm_chg_max : Outport  Port=2
  Discharge Buffer : Outport  Port=3
  Charge Buffer : Outport  Port=4
  t_coolant : Outport  Port=5
  undervolt : Outport  Port=6
  overvolt : Outport  Port=7
  tag scope: bcm_chg_max=global
  wires:
  [bcm_chg_max] -> Terminator/1
  Gain1/1 -> Derate2/3(Current Limit), To Workspace9/1
  Gain/1 -> To Workspace10/1, Derate/1(Current Limit)
  Compare To Constant1/1 -> undervolt/1
  Compare To Constant2/1 -> overvolt/1
  Constant3/1 -> t_coolant/1
  vcell/1 -> Compare To Constant2/1, Compare To Constant1/1
  Average Current/4(Charge Cont) -> Derate2/2(Cont Current)
  Average Current/3(Charge Buffer) -> Charge Buffer/1, Derate2/1(Buffer)
  Average Current/2(Discharge Cont) -> Derate/3(Cont Current)
  Average Current/1(Discharge Buffer) -> Discharge Buffer/1, Derate/2(Buffer)
  [BMS_SOC] -> bcm_chg_max_tbl/1, bcm_dis_max_tbl/1, Average Current/1(SOC)
  Derate2/1(Derate) -> bcm_chg_max/1, [bcm_chg_max], To Workspace4/1
  bcm_chg_max_tbl/1 -> Gain1/1  "bcm_chg_max"
  Derate/1(Derate) -> To Workspace3/1, bcm_dis_max/1
  bcm_dis_max_tbl/1 -> Gain/1
  [BMS_Temperatur] -> Average Current/2(Temp), bcm_dis_max_tbl/2, bcm_chg_max_tbl/2

== system lib_HVESS/ESS/Soft BMS/NMH_BMS1 ==
  Bus Creator8 : BusCreator  Inputs=5
  NMH_BMS : Outport
  wires:
  [NMH_BMS_Car_WakeUp] -> Bus Creator8/5  "NMH_BMS_Car_WakeUp"
  [NMH_BMS_Normal_Mode_1] -> Bus Creator8/1  "NMH_BMS_Normal_Mode_1"
  [NMH_BMS_Start_2] -> Bus Creator8/4  "NMH_BMS_Start_2"
  Bus Creator8/1 -> NMH_BMS/1  "NMH_BMS"
  [NMH_BMS_Normal_Mode_2] -> Bus Creator8/2  "NMH_BMS_Normal_Mode_2"
  [NMH_BMS_Start_1] -> Bus Creator8/3  "NMH_BMS_Start_1"

== system lib_HVESS/ESS/Soft BMS/NoiseAdd ==
  In : Inport
  Random Number : RandomNumber  Variance=0.1  SampleTime=tloop
  Rate Transition : RateTransition
  Sum : Sum  Inputs=|++
  Out : Outport
  wires:
  Rate Transition/1 -> Sum/2
  Sum/1 -> Out/1
  In/1 -> Sum/1
  Random Number/1 -> Rate Transition/1

== system lib_HVESS/ESS/Soft BMS/RollingAliveCnt1 ==
  Constant : Constant
  Rolling Alive Counter : Stateflow chart  TreatAsAtomicUnit=on
  Switch : Switch  Criteria=u2 > Threshold
  Out1 : Outport
  wires:
  Constant/1 -> Switch/1
  Rolling Alive Counter/1(RollingAliveCnt) -> Switch/3
  [BMS_CAN_fault] -> Switch/2
  Switch/1 -> Out1/1

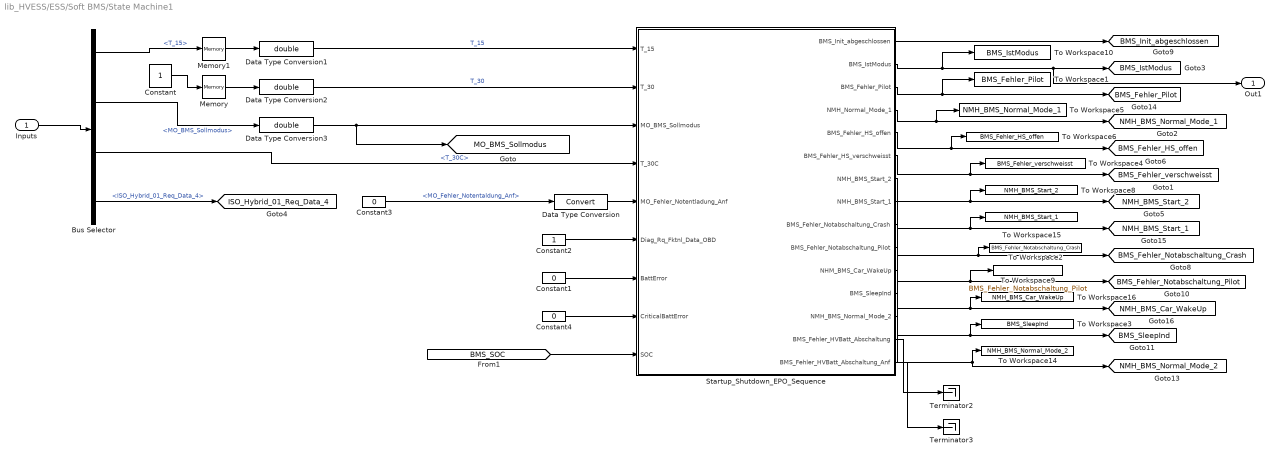
== system lib_HVESS/ESS/Soft BMS/State Machine1 ==
  Inputs : Inport
  Bus Selector : BusSelector  OutputSignals=Digital.T_15,CAN.to HV_CAN.MSG_HYB_01.MO_BMS_Sollmodus,Digital.T_30C,CAN.to EBCAN.ISO_Hybrid_01_Req.ISO_Hybrid_01_Req_Data_4
  Constant : Constant
  Constant1 : Constant  Value=0  OutDataTypeStr=boolean
  Constant2 : Constant  OutDataTypeStr=boolean
  Constant3 : Constant  Value=0  OutDataTypeStr=boolean
  Constant4 : Constant  Value=0  OutDataTypeStr=boolean
  Data Type Conversion : DataTypeConversion
  Data Type Conversion1 : DataTypeConversion  OutDataTypeStr=double
  Data Type Conversion2 : DataTypeConversion  OutDataTypeStr=double
  Data Type Conversion3 : DataTypeConversion  OutDataTypeStr=double
  Memory : Memory  InheritSampleTime=on
  Memory1 : Memory  InheritSampleTime=on
  Startup_Shutdown_EPO_Sequence : Stateflow chart  TreatAsAtomicUnit=on
  Terminator2 : Terminator
  Terminator3 : Terminator
  To Workspace1 : ToWorkspace  VariableName=BMS_Fehler_Pilot  SampleTime=-1
      settings: Decimation=WORKSPACE_DECIMATION
  To Workspace10 : ToWorkspace  VariableName=BMS_IstModus  SampleTime=-1
      settings: Decimation=WORKSPACE_DECIMATION
  To Workspace14 : ToWorkspace  VariableName=NMH_BMS_Normal_Mode_2  SampleTime=-1
      settings: Decimation=WORKSPACE_DECIMATION
  To Workspace15 : ToWorkspace  VariableName=NMH_BMS_Start_1  SampleTime=-1
      settings: Decimation=WORKSPACE_DECIMATION
  To Workspace16 : ToWorkspace  VariableName=NMH_BMS_Car_WakeUp  SampleTime=-1
      settings: Decimation=WORKSPACE_DECIMATION
  To Workspace2 : ToWorkspace  VariableName=BMS_Fehler_Notabschaltung_Crash  SampleTime=-1
      settings: Decimation=WORKSPACE_DECIMATION
  To Workspace3 : ToWorkspace  VariableName=BMS_SleepInd  SampleTime=-1
      settings: Decimation=WORKSPACE_DECIMATION
  To Workspace4 : ToWorkspace  VariableName=BMS_Fehler_verschweisst  SampleTime=-1
      settings: Decimation=WORKSPACE_DECIMATION
  To Workspace5 : ToWorkspace  VariableName=NMH_BMS_Normal_Mode_1  SampleTime=-1
      settings: Decimation=WORKSPACE_DECIMATION
  To Workspace6 : ToWorkspace  VariableName=BMS_Fehler_HS_offen  SampleTime=-1
      settings: Decimation=WORKSPACE_DECIMATION
  To Workspace8 : ToWorkspace  VariableName=NMH_BMS_Start_2  SampleTime=-1
      settings: Decimation=WORKSPACE_DECIMATION
  To Workspace9 : ToWorkspace  VariableName=BMS_Fehler_Notabschaltung_Pilot  SampleTime=-1
      settings: Decimation=WORKSPACE_DECIMATION
  Out1 : Outport
  tag scope: BMS_Fehler_HS_offen=global, BMS_Fehler_Notabschaltung_Crash=global, BMS_Fehler_Notabschaltung_Pilot=global, BMS_Fehler_Pilot=global, BMS_Fehler_verschweisst=global, BMS_Init_abgeschlossen=global, BMS_IstModus=global, BMS_SleepInd=global, ISO_Hybrid_01_Req_Data_4=global, MO_BMS_Sollmodus=global, NMH_BMS_Car_WakeUp=global, NMH_BMS_Normal_Mode_1=global, NMH_BMS_Normal_Mode_2=global, NMH_BMS_Start_1=global, NMH_BMS_Start_2=global
  wires:
  Constant/1 -> Memory/1
  [BMS_SOC] -> Startup_Shutdown_EPO_Sequence/9(SOC)
  Bus Selector/4 -> [ISO_Hybrid_01_Req_Data_4]  "<ISO_Hybrid_01_Req_Data_4>"
  Startup_Shutdown_EPO_Sequence/12(BMS_SleepInd) -> To Workspace3/1, [BMS_SleepInd]
  Startup_Shutdown_EPO_Sequence/5(BMS_Fehler_HS_offen) -> To Workspace6/1, [BMS_Fehler_HS_offen]
  Startup_Shutdown_EPO_Sequence/10(BMS_Fehler_Notabschaltung_Pilot) -> To Workspace9/1, [BMS_Fehler_Notabschaltung_Pilot]
  Startup_Shutdown_EPO_Sequence/9(BMS_Fehler_Notabschaltung_Crash) -> To Workspace2/1, [BMS_Fehler_Notabschaltung_Crash]
  Startup_Shutdown_EPO_Sequence/4(NMH_Normal_Mode_1) -> To Workspace5/1, [NMH_BMS_Normal_Mode_1]
  Startup_Shutdown_EPO_Sequence/6(BMS_Fehler_HS_verschweisst) -> [BMS_Fehler_verschweisst], To Workspace4/1
  Bus Selector/1 -> Memory1/1  "<T_15>"
  Startup_Shutdown_EPO_Sequence/2(BMS_IstModus) -> Out1/1, [BMS_IstModus], To Workspace10/1
  Startup_Shutdown_EPO_Sequence/1(BMS_Init_abgeschlossen) -> [BMS_Init_abgeschlossen]
  Startup_Shutdown_EPO_Sequence/3(BMS_Fehler_Pilot) -> To Workspace1/1, [BMS_Fehler_Pilot]
  Startup_Shutdown_EPO_Sequence/13(NMH_BMS_Normal_Mode_2) -> To Workspace14/1, [NMH_BMS_Normal_Mode_2]
  Startup_Shutdown_EPO_Sequence/7(NMH_BMS_Start_2) -> To Workspace8/1, [NMH_BMS_Start_2]
  Startup_Shutdown_EPO_Sequence/8(NMH_BMS_Start_1) -> [NMH_BMS_Start_1], To Workspace15/1
  Startup_Shutdown_EPO_Sequence/11(NHM_BMS_Car_WakeUp) -> To Workspace16/1, [NMH_BMS_Car_WakeUp]
  Bus Selector/3 -> Startup_Shutdown_EPO_Sequence/4(T_30C)  "<T_30C>"
  Constant3/1 -> Data Type Conversion/1  "<MO_Fehler_Notentaldung_Anf>"
  Constant1/1 -> Startup_Shutdown_EPO_Sequence/7(BattError)
  Constant2/1 -> Startup_Shutdown_EPO_Sequence/6(Diag_Rq_Fktnl_Data_OBD)
  Constant4/1 -> Startup_Shutdown_EPO_Sequence/8(CriticalBattError)
  Startup_Shutdown_EPO_Sequence/14(BMS_Fehler_HVBatt_Abschaltung) -> Terminator2/1
  Startup_Shutdown_EPO_Sequence/15(BMS_Fehler_HVBatt_Abschaltung_Anf) -> Terminator3/1
  Inputs/1 -> Bus Selector/1
  Bus Selector/2 -> Data Type Conversion3/1  "<MO_BMS_Sollmodus>"
  Data Type Conversion/1 -> Startup_Shutdown_EPO_Sequence/5(MO_Fehler_Notentladung_Anf)
  Data Type Conversion1/1 -> Startup_Shutdown_EPO_Sequence/1(T_15)  "T_15"
  Data Type Conversion2/1 -> Startup_Shutdown_EPO_Sequence/2(T_30)  "T_30"
  Memory/1 -> Data Type Conversion2/1
  Memory1/1 -> Data Type Conversion1/1
  Data Type Conversion3/1 -> Startup_Shutdown_EPO_Sequence/3(MO_BMS_Sollmodus), [MO_BMS_Sollmodus]

== system lib_HVESS/ESS/Soft BMS/Temperature Management ==
  ess_temp : Inport
  Add2 : Sum  Inputs=+-
  Constant : Constant
  Constant1 : Constant  Value=3
  Constant2 : Constant  Commented=on  Value=BMS_Notfallkuehlung
  Constant3 : Constant
  K : Constant  Value=273.15
  Switch : Switch
  tag scope: BMS_HYB_Kuehlung_Anf=global, BMS_Notfallkuehlung=global, BMS_Temperatur=global, BMS_Temperierung_Anf=global
  wires:
  Add2/1 -> [BMS_Temperatur]
  K/1 -> Add2/2
  ess_temp/1 -> Switch/2, Add2/1
  Constant3/1 -> [BMS_Notfallkuehlung]
  Constant1/1 -> Switch/3
  Switch/1 -> [BMS_Temperierung_Anf], [BMS_HYB_Kuehlung_Anf]
  Constant/1 -> Switch/1

== system lib_HVESS/ESS/ESS/Bosch_Li_Cell/Subsystem ==
  In1 : Inport
  In2 : Inport  Port=2
  Gain3 : Gain  Gain=I_loss
  Memory : Memory  InheritSampleTime=on
  Relational Operator : RelationalOperator  Operator=>  OutDataTypeStr=boolean  RndMeth=Nearest
  Switch : Switch  Criteria=u2 > Threshold
  Out1 : Outport
  wires:
  Memory/1 -> Switch/1, Relational Operator/1
  Switch/1 -> Out1/1
  Relational Operator/1 -> Switch/2
  In1/1 -> Memory/1
  In2/1 -> Gain3/1
  Gain3/1 -> Switch/3, Relational Operator/2

== system lib_HVESS/ESS/ESS/Cooling_Loop1/Sensor ==
  Ideal Temperature Sensor : fl_lib/Thermal/Thermal Sensors/Temperature Sensor
  PS-Simulink Converter : nesl_utility/PS-Simulink Converter  PhysicalDomain=network_engine_domain  SubClassName=ps_output  LeftPortType=input  RightPortType=output  PseudoPeriodic=off  Frequencies=[]  Unit=1  AffineConversion=off
  Scope : Scope
  Thermal Reference : fl_lib/Thermal/Thermal Elements/Thermal Reference
  B : PMIOPort  Port=1  Side=Left
  wires:
  PS-Simulink Converter/1 -> Scope/1
  connections:
  PS-Simulink Converter/LConn1 -- Ideal Temperature Sensor/RConn2
  Ideal Temperature Sensor/RConn1 -- Thermal Reference/LConn1
  B/RConn1 -- Ideal Temperature Sensor/LConn1

== system lib_HVESS/ESS/Soft BMS/BMS_HYB_1/BMS_HYB_02_BZ ==
  Constant : Constant
  Constant1 : Constant  Value=0
  Rolling Alive Counter1 : RollingAliveCounter/Rolling Alive Counter
      settings: SourceProductName=The database C:\Users\vrajm\AppData\Roaming\MathWorks\MATLAB\R2017b\slblocks_master.db is locked, or a table in the database is locked. (database is locked)
  Switch : Switch  Criteria=u2 > Threshold
  Out1 : Outport
  tag scope: BMS_CAN_fault=global
  wires:
  Constant1/1 -> [BMS_CAN_fault]
  Switch/1 -> Out1/1  "BMS_HYB_02_BZ"
  Rolling Alive Counter1/1 -> Switch/3
  Constant/1 -> Switch/1
  [BMS_CAN_fault] -> Switch/2

== system lib_HVESS/ESS/Soft BMS/Energy Consumption/Divide by zero ==
  In1 : Inport
  Compare To Constant : simulink/Logic and Bit Operations/Compare To Constant  relop===  const=0  OutDataTypeStr=boolean
  Constant1 : Constant  Value=eps
  Switch2 : Switch  Criteria=u2 > Threshold
  Out1 : Outport
  wires:
  Switch2/1 -> Out1/1
  In1/1 -> Compare To Constant/1, Switch2/3
  Compare To Constant/1 -> Switch2/2
  Constant1/1 -> Switch2/1

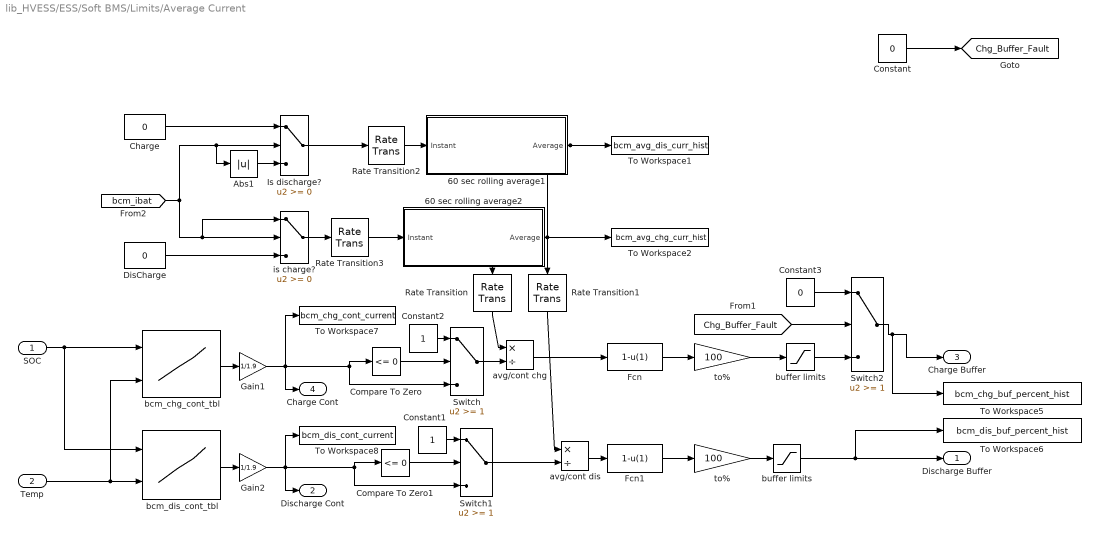
== system lib_HVESS/ESS/Soft BMS/Limits/Average Current ==
  SOC : Inport
  Temp : Inport  Port=2
  60 sec rolling average1 : Subsystem
  60 sec rolling average2 : Subsystem
  Abs1 : Abs
  Charge : Constant  Value=0
  Compare To Zero : simulink/Logic and Bit Operations/Compare To Zero  relop=<=  OutDataTypeStr=boolean
  Compare To Zero1 : simulink/Logic and Bit Operations/Compare To Zero  relop=<=  OutDataTypeStr=boolean
  Constant : Constant  Value=0
  Constant1 : Constant
  Constant2 : Constant
  Constant3 : Constant  Value=0
  DisCharge : Constant  Value=0
  Fcn : Fcn  Expr=1-u(1)
  Fcn1 : Fcn  Expr=1-u(1)
  Gain1 : Gain  Gain=1/1.9
  Gain2 : Gain  Gain=1/1.9
  Is discharge? : Switch
  Rate Transition{,1..3} (4 alike) : RateTransition
  Switch : Switch  Threshold=1
  Switch1 : Switch  Threshold=1
  Switch2 : Switch  Threshold=1
  To Workspace1 : ToWorkspace  VariableName=bcm_avg_dis_curr_hist  SampleTime=-1
      settings: Decimation=WORKSPACE_DECIMATION
  To Workspace2 : ToWorkspace  VariableName=bcm_avg_chg_curr_hist  SampleTime=-1
      settings: Decimation=WORKSPACE_DECIMATION
  To Workspace5 : ToWorkspace  VariableName=bcm_chg_buf_percent_hist  SampleTime=-1
      settings: Decimation=WORKSPACE_DECIMATION
  To Workspace6 : ToWorkspace  VariableName=bcm_dis_buf_percent_hist  SampleTime=-1
      settings: Decimation=WORKSPACE_DECIMATION
  To Workspace7 : ToWorkspace  VariableName=bcm_chg_cont_current  SampleTime=-1
      settings: Decimation=WORKSPACE_DECIMATION
  To Workspace8 : ToWorkspace  VariableName=bcm_dis_cont_current  SampleTime=-1
      settings: Decimation=WORKSPACE_DECIMATION
  avg/cont chg : Product  Inputs=*/  RndMeth=Zero
  avg/cont dis : Product  Inputs=*/  RndMeth=Zero
  bcm_chg_cont_tbl : Lookup2D  RowIndex=ess.plant.init.limit.idx1_soc  ColumnIndex=ess.plant.init.limit.idx2_temp  Table=ess.plant.init.max_cont_charge
  bcm_dis_cont_tbl : Lookup2D  RowIndex=ess.plant.init.limit.idx1_soc  ColumnIndex=ess.plant.init.limit.idx2_temp  Table=ess.plant.init.max_cont_discharge
  buffer limits : Saturate  UpperLimit=100  LowerLimit=0
  "buffer limits " : Saturate  UpperLimit=100  LowerLimit=0
  is charge? : Switch
  to% : Gain  Gain=100
  "to% " : Gain  Gain=100
  Discharge Buffer : Outport
  Discharge Cont : Outport  Port=2
  Charge Buffer : Outport  Port=3
  Charge Cont : Outport  Port=4
  tag scope: Chg_Buffer_Fault=global
  wires:
  Constant/1 -> [Chg_Buffer_Fault]
  Rate Transition3/1 -> 60 sec rolling average2/1(Instant)
  Rate Transition2/1 -> 60 sec rolling average1/1(Instant)
  Rate Transition1/1 -> avg/cont dis/1
  Rate Transition/1 -> avg/cont chg/1
  Gain2/1 -> To Workspace8/1, Switch1/3, Compare To Zero1/1, Discharge Cont/1
  Gain1/1 -> Charge Cont/1, Switch/3, Compare To Zero/1, To Workspace7/1
  "buffer limits "/1 -> Discharge Buffer/1, To Workspace6/1
  bcm_dis_cont_tbl/1 -> Gain2/1
  Switch1/1 -> avg/cont dis/2
  Constant1/1 -> Switch1/1
  Compare To Zero1/1 -> Switch1/2
  bcm_chg_cont_tbl/1 -> Gain1/1
  Switch/1 -> avg/cont chg/2
  Constant2/1 -> Switch/1
  Compare To Zero/1 -> Switch/2
  SOC/1 -> bcm_dis_cont_tbl/1, bcm_chg_cont_tbl/1
  [bcm_ibat] -> Is discharge?/2, Abs1/1, is charge?/2, is charge?/1
  Charge/1 -> Is discharge?/1
  Abs1/1 -> Is discharge?/3
  DisCharge/1 -> is charge?/3
  Is discharge?/1 -> Rate Transition2/1
  is charge?/1 -> Rate Transition3/1
  60 sec rolling average1/1(Average) -> To Workspace1/1, Rate Transition1/1
  60 sec rolling average2/1(Average) -> To Workspace2/1, Rate Transition/1
  avg/cont chg/1 -> Fcn/1
  avg/cont dis/1 -> Fcn1/1
  Fcn/1 -> to%/1
  Fcn1/1 -> "to% "/1
  "to% "/1 -> "buffer limits "/1
  to%/1 -> buffer limits/1
  Temp/1 -> bcm_chg_cont_tbl/2, bcm_dis_cont_tbl/2
  buffer limits/1 -> Switch2/3
  Switch2/1 -> Charge Buffer/1, To Workspace5/1
  Constant3/1 -> Switch2/1
  [Chg_Buffer_Fault] -> Switch2/2

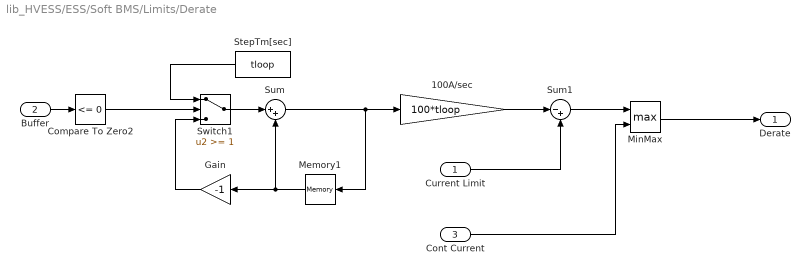
== system lib_HVESS/ESS/Soft BMS/Limits/Derate ==
  Current Limit : Inport
  Buffer : Inport  Port=2
  Cont Current : Inport  Port=3
  100A/sec : Gain  Gain=100*tloop
  Compare To Zero2 : simulink/Logic and Bit Operations/Compare To Zero  relop=<=  OutDataTypeStr=boolean
  Gain : Gain  Gain=-1
  Memory1 : Memory
  MinMax : MinMax  Function=max  Inputs=2
  StepTm[sec] : Constant  Value=tloop
  Sum : Sum  Inputs=|++
  Sum1 : Sum  Inputs=|-+
  Switch1 : Switch  Threshold=1
  Derate : Outport
  wires:
  Cont Current/1 -> MinMax/2
  MinMax/1 -> Derate/1
  Current Limit/1 -> Sum1/2
  Sum1/1 -> MinMax/1
  100A/sec/1 -> Sum1/1
  Compare To Zero2/1 -> Switch1/2
  Buffer/1 -> Compare To Zero2/1
  Gain/1 -> Switch1/3
  Memory1/1 -> Sum/2, Gain/1
  StepTm[sec]/1 -> Switch1/1
  Switch1/1 -> Sum/1
  Sum/1 -> 100A/sec/1, Memory1/1

== system lib_HVESS/ESS/Soft BMS/Limits/Derate2 ==
  Buffer : Inport
  Cont Current : Inport  Port=2
  Current Limit : Inport  Port=3
  100A/sec : Gain  Gain=100*tloop
  Compare To Zero2 : simulink/Logic and Bit Operations/Compare To Zero  relop=<=  OutDataTypeStr=boolean
  Gain : Gain  Gain=-1
  Memory1 : Memory
  MinMax : MinMax  Function=max  Inputs=2
  StepTm[sec] : Constant  Value=tloop
  Sum : Sum  Inputs=|++
  Sum1 : Sum  Inputs=|-+
  Switch1 : Switch  Threshold=1
  Derate : Outport
  wires:
  Sum/1 -> Memory1/1, 100A/sec/1
  Switch1/1 -> Sum/1
  StepTm[sec]/1 -> Switch1/1
  Memory1/1 -> Gain/1, Sum/2
  Gain/1 -> Switch1/3
  Buffer/1 -> Compare To Zero2/1
  Compare To Zero2/1 -> Switch1/2
  100A/sec/1 -> Sum1/1
  Sum1/1 -> MinMax/1
  Current Limit/1 -> Sum1/2
  MinMax/1 -> Derate/1
  Cont Current/1 -> MinMax/2

== system lib_HVESS/ESS/Soft BMS/Limits/Average Current/60 sec rolling average1 ==
  Instant : Inport
  1 second : Delay  DelayLength=1/tloop  InputProcessing=Inherited  SampleTime=tloop
  1sec trigger : Subsystem
  60 sec average : Subsystem
  Gain1 : Gain  Gain=tloop
  Rate Transition : RateTransition
  Sum1 : Sum  Inputs=++-
  accumulate : Memory  InheritSampleTime=on
  accumulate1 : Memory  InheritSampleTime=on
  Average : Outport
  wires:
  Rate Transition/1 -> 60 sec average/1(1sec)
  Gain1/1 -> Rate Transition/1
  1sec trigger/1(Trigger) -> 60 sec average/Enable
  Sum1/1 -> accumulate/1, Gain1/1
  Instant/1 -> 1 second/1, Sum1/2
  1 second/1 -> Sum1/3
  accumulate/1 -> Sum1/1
  60 sec average/1(Average) -> accumulate1/1
  accumulate1/1 -> Average/1

== system lib_HVESS/ESS/Soft BMS/Limits/Average Current/60 sec rolling average2 ==
  Instant : Inport
  1 second : Delay  DelayLength=1/tloop  InputProcessing=Inherited  SampleTime=tloop
  1sec trigger : Subsystem
  60 sec average : Subsystem
  Gain1 : Gain  Gain=tloop
  Rate Transition : RateTransition
  Sum1 : Sum  Inputs=++-
  accumulate : Memory  InheritSampleTime=on
  accumulate1 : Memory  InheritSampleTime=on
  Average : Outport
  wires:
  Rate Transition/1 -> 60 sec average/1(1sec)
  Gain1/1 -> Rate Transition/1
  1sec trigger/1(Trigger) -> 60 sec average/Enable
  accumulate1/1 -> Average/1
  60 sec average/1(Average) -> accumulate1/1
  accumulate/1 -> Sum1/1
  1 second/1 -> Sum1/3
  Instant/1 -> Sum1/2, 1 second/1
  Sum1/1 -> Gain1/1, accumulate/1

== system lib_HVESS/ESS/Soft BMS/Limits/Average Current/60 sec rolling average1/1sec trigger ==
  0 : Constant  Value=0
  Compare To Constant : simulink/Logic and Bit Operations/Compare To Constant  relop=<=  const=3.0  OutDataTypeStr=boolean
  Data Type Conversion : DataTypeConversion
  Sum2 : Sum  Inputs=|++
  Switch : Switch  Threshold=0.5
  accumulate2 : Memory  InheritSampleTime=on
  tloop : Constant  Value=tloop
  Trigger : Outport
  wires:
  tloop/1 -> Sum2/1
  accumulate2/1 -> Sum2/2
  Sum2/1 -> Compare To Constant/1, Switch/3
  Switch/1 -> accumulate2/1
  Compare To Constant/1 -> Data Type Conversion/1
  0/1 -> Switch/1
  Data Type Conversion/1 -> Switch/2, Trigger/1

== system lib_HVESS/ESS/Soft BMS/Limits/Average Current/60 sec rolling average1/60 sec average ==
  1sec : Inport
  Enable : EnablePort
  60 second : Delay  DelayLength=60  InputProcessing=Inherited  SampleTime=tloop
  Gain2 : Gain  Gain=1/60
  Sum2 : Sum  Inputs=++-
  accumulate2 : Memory  InheritSampleTime=on
  Average : Outport
  wires:
  Sum2/1 -> accumulate2/1, Gain2/1
  60 second/1 -> Sum2/3
  accumulate2/1 -> Sum2/1
  Gain2/1 -> Average/1
  1sec/1 -> 60 second/1, Sum2/2

== system lib_HVESS/ESS/Soft BMS/Limits/Average Current/60 sec rolling average2/1sec trigger ==
  0 : Constant  Value=0
  Compare To Constant : simulink/Logic and Bit Operations/Compare To Constant  relop=<=  const=3.0  OutDataTypeStr=boolean
  Data Type Conversion : DataTypeConversion
  Sum2 : Sum  Inputs=|++
  Switch : Switch  Threshold=0.5
  accumulate2 : Memory  InheritSampleTime=on
  tloop : Constant  Value=tloop
  Trigger : Outport
  wires:
  tloop/1 -> Sum2/1
  accumulate2/1 -> Sum2/2
  Sum2/1 -> Compare To Constant/1, Switch/3
  Switch/1 -> accumulate2/1
  Compare To Constant/1 -> Data Type Conversion/1
  0/1 -> Switch/1
  Data Type Conversion/1 -> Switch/2, Trigger/1

== system lib_HVESS/ESS/Soft BMS/Limits/Average Current/60 sec rolling average2/60 sec average ==
  1sec : Inport
  Enable : EnablePort
  60 second : Delay  DelayLength=60  InputProcessing=Inherited  SampleTime=tloop
  Gain2 : Gain  Gain=1/60
  Sum2 : Sum  Inputs=++-
  accumulate2 : Memory  InheritSampleTime=on
  Average : Outport
  wires:
  Sum2/1 -> accumulate2/1, Gain2/1
  60 second/1 -> Sum2/3
  accumulate2/1 -> Sum2/1
  Gain2/1 -> Average/1
  1sec/1 -> 60 second/1, Sum2/2

== stateflow chart lib_HVESS/ESS/Soft BMS/RollingAliveCnt1/Rolling Alive Counter ==
  state RollingAliveCounter
    state Count1
      en: RollingAliveCnt = 0;
    state Count2
      en: RollingAliveCnt = 1;
    state Count3
      en: RollingAliveCnt = 2;
    state Count4
      en: RollingAliveCnt = 3;
    (default) -> Count1
    Count4 -> Count1 : after(0.01,sec)
    Count1 -> Count2 : after(0.01,sec)
    Count2 -> Count3 : after(0.01,sec)
    Count3 -> Count4 : after(0.01,sec)
  data: RollingAliveCnt output int8 =0
